simulink model "pid_discrete_antiwindup"  (R2018b)
settings: Solver=ode45  StartTime=0.0  StopTime=10  FixedStep=0.05  RelTol=1e-3
values from neighbouring files (symbols this model uses):
  A = [-b/J   K/J ... (first row only)    [motor_model.m]
  B = [0 ... (first row only)    [motor_model.m]
  C = [1   0]    [motor_model.m]
  D = 0    [motor_model.m]
settings Model: Creator=kika  LastModifiedBy=kika
settings DataIOCC: ReturnWorkspaceOutputs=on

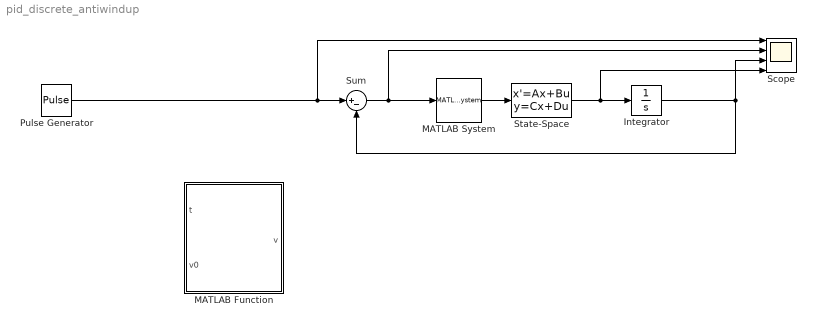
== system pid_discrete_antiwindup ==
  Integrator : Integrator
  MATLAB Function : MATLAB Function  TreatAsAtomicUnit=on
  MATLAB System : MATLABSystem  System=PID  kp=10  ki=0  kd=0  dt=0.0005  kt=0  u_max=10  u_min=-10  SimulateUsing=Interpreted execution
      mask Type: PID
      mask Display:
      | disp('PID');
      | port_label('input',1,'e');
      | port_label('output',1,'y');
  Pulse Generator : DiscretePulseGenerator  PulseType=Time based  Period=5  PulseWidth=50  PhaseDelay=0.5
  Scope : Scope  NumInputPorts=4
  State-Space : StateSpace  A=A  B=B  C=C  D=D  InitialCondition=[0,0]'
  Sum : Sum  Inputs=|+-
  wires:
  MATLAB System/1 -> State-Space/1
  Sum/1 -> Scope/2, MATLAB System/1
  Pulse Generator/1 -> Scope/1, Sum/1
  State-Space/1 -> Scope/4, Integrator/1
  Integrator/1 -> Sum/2, Scope/3

== matlab function pid_discrete_antiwindup/MATLAB Function ==
  data: t input; v0 input; v output
function v = ramp(t, v0)

    a = 2;
    v = v0 + a * t;
    

%     t1 = 1.5 * (q1 - q0) / v;
%     tb = (q0 - q1 + v * t1) / v;
%     a = v / tb;
% 
%     if t <= tb
%         % initial blend
%         p = q0 + a/2*tt^2;
%         pd = a*tt;
%         pdd = a;
%     elseif t <= (t1 - tb)
%         % linear motion
%         p = (q1+q0-V*tf)/2 + V*tt;
%         pd = V;
%         pdd = 0;
%     else
%         % final blend
%         p = q1 - a/2*tf^2 + a*tf*tt - a/2*tt^2;
%         pd = a*tf - a*tt;
%         pdd = -a;
%     end
